simulink model "AdaptiveIDMF"  (R2022a)
settings: Solver=ode4  StartTime=0.0  StopTime=30  FixedStep=0.01  RelTol=1e-3
PostLoadFcn:
  | %Add subfolders to path
  | addpath('virtualworld');
InitFcn:
  | startScript;
values from neighbouring files (symbols this model uses):
  angularVelocity = [0 0 -0.01]    [startScript.m]
  angularVelocityforLanding = [0 0 0]    [startScript.m]
  dronestartlocation = [-1.5 0 4]    [startScript.m]
  Dstar = -0.5    [startScript.m]
  finalHoverHeight = 2.5    [startScript.m]
  helipadLocation = [14 0.6 5]    [startScript.m]
  linearVelocity = [5 0.05 1]    [startScript.m]
  linearVelocityforHover = [0.65 0.05 0.3]    [startScript.m]
  ypmin = yps(iypmin,:)    [hyperpred.m]
undefined symbols (not defined in the file or in its folder): fspecial, gcbh, Kanade, Lucas, Rec, SDTV, vrmfunc
libraries: visiontextngfix x10, visionconversions x9, vrlib x7, visionanalysis x7, slpidlib x4, sharedtransform x2, simulink x1
(part 2 of 3)

== system AdaptiveIDMF/ Optical Flow Algorithm for Obstacle Avoidance/Optical flow algorithm and PID Controller for landing/DronePositionEstimation.OpticalFlowAlgorithm_ ==
  note: If the output from the Sign block is Positive, drone should move towards the left side, i.e. V_y is Negative. Also, if the output from the Sign block is Negative, drone will move towwars the right side..ie, V_y is Positive.
  note: Steering Linear Velocities
  OpticalFlowDiff : Inport
  Action Port : ActionPort
      settings: CopyFcn=Stateflow.SLINSF.SimulinkMan.removeBlockPreDeleteFcn  PreDeleteFcn=Stateflow.SLINSF.SimulinkMan.unsafePredeleteFcn
  Constant : Constant  Value=uint32(zeros(50,2))
  Constant1 : Constant  Value=linearVelocity
  Constant3 : Constant  Value=-1
  Gain : Gain  Gain=[1 1 -1]
  Integrator2 : Integrator  InitialCondition=dronestartlocation
  Sign : Signum
  Switch1 : Switch  Criteria=u2 > Threshold  SaturateOnIntegerOverflow=off  InputSameDT=off
  PositionOutput : Outport
  detectedpoints : Outport  Port=2
      settings: VarSizeSig=Yes
  reset : Outport  Port=3
  wires:
  OpticalFlowDiff/1 -> Sign/1
  Constant1/1 -> Switch1/3, Gain/1  "[V_X V_Z V_Y]"
  Switch1/1 -> Integrator2/1
  Gain/1 -> Switch1/1  "[V_X V_Z -1*V_Y]"
  Constant/1 -> detectedpoints/1
  Sign/1 -> Switch1/2
  Integrator2/1 -> PositionOutput/1
  Constant3/1 -> reset/1

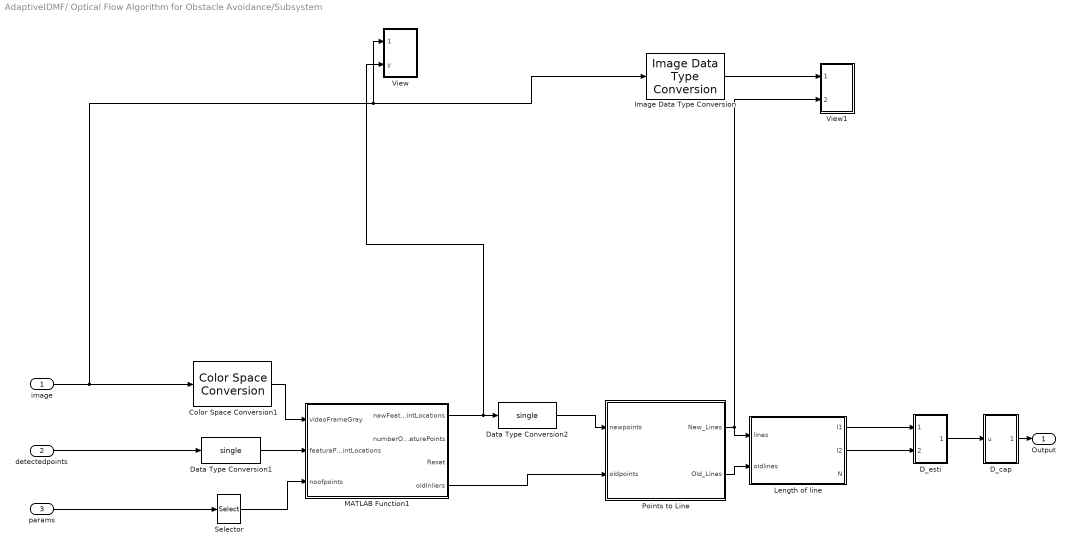
== system AdaptiveIDMF/ Optical Flow Algorithm for Obstacle Avoidance/Subsystem ==
  image : Inport
  detectedpoints : Inport  Port=2
  params : Inport  Port=3
  Color Space Conversion1 : visionconversions/Color Space  Conversion  conversion=Obsolete  conversionActive=R'G'B' to intensity  wp_str=D65  rec=Rec. 601 (SDTV)  sys=1125/60/2:1  imagePorts=One multidimensional signal
  D_cap : Subsystem
  D_esti : Subsystem
  Data Type Conversion1 : DataTypeConversion  OutDataTypeStr=single  SaturateOnIntegerOverflow=off  RndMeth=Floor
  Data Type Conversion2 : DataTypeConversion  OutDataTypeStr=single  SaturateOnIntegerOverflow=off  RndMeth=Floor
  Image Data Type Conversion : visionconversions/Image Data Type Conversion  outDT=single  isSigned=on  wordLen=16  numFracBits=0
      settings: SourceProductBaseCode=VP
  Length of line : MATLAB Function  TreatAsAtomicUnit=on
  MATLAB Function1 : MATLAB Function  TreatAsAtomicUnit=on
  Points to Line : MATLAB Function  TreatAsAtomicUnit=on
  Selector : Selector  InputPortWidth=6  IndexOptions=Index vector (dialog)  Indices=2  OutputSizes=1
  View : Subsystem
  View1 : Subsystem
  Output : Outport
  wires:
  Data Type Conversion1/1 -> MATLAB Function1/2(featurePointLocations)
  Color Space Conversion1/1 -> MATLAB Function1/1(videoFrameGray)
  MATLAB Function1/4(oldInliers) -> Points to Line/2(oldpoints)
  Points to Line/2(Old_Lines) -> Length of line/2(oldlines)
  params/1 -> Selector/1
  Selector/1 -> MATLAB Function1/3(noofpoints)
  Length of line/1(l1) -> D_esti/1(In1)
  Length of line/2(l2) -> D_esti/2(In2)
  D_esti/1(Out1) -> D_cap/1(u)
  D_cap/1(Out1) -> Output/1
  MATLAB Function1/1(newFeaturePointLocations) -> View/2(y), Data Type Conversion2/1
  Data Type Conversion2/1 -> Points to Line/1(newpoints)
  detectedpoints/1 -> Data Type Conversion1/1
  image/1 -> Image Data Type Conversion/1, View/1(d_camera), Color Space Conversion1/1
  Points to Line/1(New_Lines) -> View1/2(vel_Lines), Length of line/1(lines)
  Image Data Type Conversion/1 -> View1/1(camera_d)

== system AdaptiveIDMF/ Optical Flow Algorithm for Obstacle Avoidance/flowdiff ==
  image : Inport
  Delay1 : Delay  DelayLength=4
  FlowDifferences : MATLAB Function  TreatAsAtomicUnit=on
  Gain : Gain  Gain=1/10^3
  Sum1 : Sum  Inputs=+-
  Out1 : Outport
  Out2 : Outport  Port=2
  vleftflow : Outport  Port=3
  vrightflow : Outport  Port=4
  cmd : Outport  Port=5
  wires:
  Gain/1 -> Out2/1, Delay1/1, Sum1/1
  FlowDifferences/1(flowDifference) -> Gain/1
  Sum1/1 -> Out1/1
  FlowDifferences/3(vrightflow) -> vrightflow/1
  FlowDifferences/4(cmd) -> cmd/1
  Delay1/1 -> Sum1/2
  image/1 -> FlowDifferences/1(image)
  FlowDifferences/2(vleftflow) -> vleftflow/1

== system AdaptiveIDMF/ Optical Flow Algorithm for Obstacle Avoidance/flowdiff_down ==
  image : Inport
  Delay : Delay  DelayLength=10
  Delay2 : Delay  DelayLength=10
  FlowDifferences1 : MATLAB Function  TreatAsAtomicUnit=on
  FlowDifferences2 : MATLAB Function  TreatAsAtomicUnit=on
  Gain1 : Gain  Gain=1/10^3
  Gain2 : Gain  Gain=1/10^3
  Sum : Sum  Inputs=+-
  Sum2 : Sum  Inputs=+-
  ofd_up_d : Outport
  flowdiff_down : Outport  Port=2
  ofd_d : Outport  Port=3
  flowup_down : Outport  Port=4
  wires:
  image/1 -> FlowDifferences2/1(image), FlowDifferences1/1(image)
  Gain1/1 -> flowdiff_down/1, Sum/1, Delay/1  "flowdiff_down"
  Gain2/1 -> flowup_down/1, Delay2/1, Sum2/1  "flowup_down"
  FlowDifferences1/1(flowDifference) -> Gain1/1  "flowdiff_down"
  Delay/1 -> Sum/2
  FlowDifferences2/1(flowDifference) -> Gain2/1  "flowup_down"
  Sum2/1 -> ofd_up_d/1  "ofd_up_d"
  Delay2/1 -> Sum2/2
  Sum/1 -> ofd_d/1  "ofd_d"

== system AdaptiveIDMF/Optical Flow Lines Calculation/Optical Flow Lines ==
  vel.Values : Inport
  Optical Flow Lines : MATLAB Function  TreatAsAtomicUnit=on
  vel.Lines : Outport
  wires:
  Optical Flow Lines/1(vel_Lines) -> vel.Lines/1
  vel.Values/1 -> Optical Flow Lines/1(vel_Values)

== system AdaptiveIDMF/Optical Flow Lines Calculation/Optical Flow Lines1 ==
  vel.Values : Inport
  Optical Flow Lines : MATLAB Function  TreatAsAtomicUnit=on
  vel.Lines : Outport
  wires:
  Optical Flow Lines/1(vel_Lines) -> vel.Lines/1
  vel.Values/1 -> Optical Flow Lines/1(vel_Values)

== system AdaptiveIDMF/Optical Flow Lines Calculation1/D ==
  Clock : Clock
  Gain : Gain  Gain=5
  Memory : Memory
  Sum1 : Sum  Inputs=+-
  Out2 : Outport
  wires:
  Clock/1 -> Memory/1, Sum1/1
  Sum1/1 -> Gain/1
  Memory/1 -> Sum1/2
  Gain/1 -> Out2/1

== system AdaptiveIDMF/Optical Flow Lines Calculation1/View ==
  d_camera : Inport
  In2 : Inport  Port=2
  Data Type Conversion : DataTypeConversion  OutDataTypeStr=int32  SaturateOnIntegerOverflow=off  RndMeth=Floor
  Draw Markers1 : visiontextngfix/Draw Markers  shape=X-mark  size=3  fill=off  fillClrSource=Specify via dialog  display=User-specified value  intensity=200  color=[255 0 0]  opacity=0.6  viewport=Entire image  antialiasing=off  inType=Obsolete  imagePorts=One multidimensional signal  roundingMode=Floor  overflowMode=off  memoryMode=Specify word length  memoryWordLength=16  memoryFracLength=15  prodOutputMode=Binary point scaling  prodOutputWordLength=32  prodOutputFracLength=14
      settings: SourceProductBaseCode=VP
  points for ownline : VideoViewer  FigPos=[132 616 560 453]
  wires:
  In2/1 -> Data Type Conversion/1
  Draw Markers1/1 -> points for ownline/1
  d_camera/1 -> Draw Markers1/1
  Data Type Conversion/1 -> Draw Markers1/2

== system AdaptiveIDMF/Optical Flow Lines Calculation1/View1 ==
  In1 : Inport
  In2 : Inport  Port=2
  Data Type Conversion : DataTypeConversion  OutDataTypeStr=int32  SaturateOnIntegerOverflow=off  RndMeth=Floor
  Draw Shapes2 : visiontextngfix/Draw Shapes  shape=Lines  fill=off  lineWidth=1  fillClrSource=Specify via dialog  display=User-specified value  intensity=200  color=[255 255 0]  opacity=0.6  viewport=Entire image  antialiasing=off  inType=Obsolete  imagePorts=One multidimensional signal  roundingMode=Floor  overflowMode=off  memoryMode=Specify word length  memoryWordLength=16  prodOutputMode=Binary point scaling  prodOutputWordLength=32  prodOutputFracLength=14  memoryFracLength=15
  owncode lines : VideoViewer  FigPos=[594 703 418 304]
  wires:
  Draw Shapes2/1 -> owncode lines/1
  In1/1 -> Draw Shapes2/1
  Data Type Conversion/1 -> Draw Shapes2/2
  In2/1 -> Data Type Conversion/1

== system AdaptiveIDMF/ Optical Flow Algorithm for Obstacle Avoidance/Optical flow algorithm and PID Controller for landing/DronePositionEstimation.DroneLandingnoZ/Landing ==
  note: Steering Linear Velocities
  In1 : Inport
  D_est : Inport  Port=2
  linearVelocity : Inport  Port=3
  ypmin : Inport  Port=4
  Bus Creator1 : BusCreator  Inputs=3
  Constant : Constant  Value=linearVelocity
  Integrator2 : Integrator  InitialConditionSource=external  InitialCondition=dronestartlocation
  Manual Switch : ManualSwitch  CurrentSetting=0
  Manual Switch1 : ManualSwitch  CurrentSetting=0
  Selector2 : Selector  InputPortWidth=3  IndexOptions=Index vector (dialog)  Indices=[2]  OutputSizes=1
  Selector3 : Selector  InputPortWidth=3  IndexOptions=Index vector (dialog)  Indices=[3]  OutputSizes=1
  Selector4 : Selector  InputPortWidth=3  IndexOptions=Index vector (dialog)  Indices=[1]  OutputSizes=1
  Subsystem : Subsystem
  PositionOutput : Outport
  reset : Outport  Port=2
  wires:
  D_est/1 -> Subsystem/2(D_est)
  Selector4/1 -> Bus Creator1/1
  Selector3/1 -> Bus Creator1/3
  Subsystem/1(Z) -> Bus Creator1/2
  Bus Creator1/1 -> PositionOutput/1
  Selector2/1 -> Subsystem/1(InitialZ)
  Manual Switch/1 -> Integrator2/1  "[V_X V_Z -1*V_Y]"
  Constant/1 -> Manual Switch/1
  Integrator2/1 -> Manual Switch1/1
  linearVelocity/1 -> Manual Switch/2
  Manual Switch1/1 -> Selector4/1, Selector3/1, Selector2/1
  In1/1 -> Integrator2/2, Manual Switch1/2
  Subsystem/2(Output) -> reset/1
  ypmin/1 -> Subsystem/3(params)

== system AdaptiveIDMF/ Optical Flow Algorithm for Obstacle Avoidance/Optical flow algorithm and PID Controller for landing/DronePositionEstimation.DroneLandingnoZ/Subsystem ==
  Input : Inport
  Color Space Conversion1 : visionconversions/Color Space  Conversion  conversion=Obsolete  conversionActive=R'G'B' to intensity  wp_str=D65  rec=Rec. 601 (SDTV)  sys=1125/60/2:1  imagePorts=One multidimensional signal
  Corner Detection : visionanalysis/Corner Detection  method=Local intensity comparison (Rosen & Drummond)  factor=0.04  filter=fspecial('gaussian', [1 5], 1.5)  thrInten=0.1  thrAngle=157.5  output=Obsolete9b  outputInUse=Corner location  maxNum=50  thrMetric=0.005  neighborSize=[15 15]  isOutVarDim=off  roundingMode=Floor  overflowMode=off  firstCoeffMode=Specify word length  firstCoeffWordLength=16  firstCoeffFracLength=16  prodOutputMode=Binary point scaling  prodOutputWordLength=32  prodOutputFracLength=0  accumMode=Binary point scaling  accumWordLength=32  accumFracLength=0  memoryMode=Binary point scaling  memoryWordLength=32  memoryFracLength=0
      settings: SourceProductBaseCode=VP
  Output : Outport
  wires:
  Input/1 -> Color Space Conversion1/1
  Color Space Conversion1/1 -> Corner Detection/1
  Corner Detection/1 -> Output/1

== system AdaptiveIDMF/ Optical Flow Algorithm for Obstacle Avoidance/Subsystem/D_cap ==
  u : Inport
  Divide1 : Product  Inputs=*/
  Pre-proessing : Subsystem
  sumele : MATLAB Function  TreatAsAtomicUnit=on
  Out1 : Outport
  wires:
  sumele/2(n1) -> Divide1/2
  Divide1/1 -> Pre-proessing/1(Dca)  "Dca"
  sumele/1(y1) -> Divide1/1
  Pre-proessing/1(Out1) -> Out1/1
  u/1 -> sumele/1(u)

== system AdaptiveIDMF/ Optical Flow Algorithm for Obstacle Avoidance/Subsystem/D_esti ==
  In1 : Inport
  In2 : Inport  Port=2
  Constant : Constant  Value=0.1
  Divide : Product  Inputs=*//
  Sum : Sum  Inputs=|-+
  Out1 : Outport
  wires:
  Sum/1 -> Divide/1
  Constant/1 -> Divide/3
  In2/1 -> Divide/2, Sum/2
  In1/1 -> Sum/1
  Divide/1 -> Out1/1

== system AdaptiveIDMF/ Optical Flow Algorithm for Obstacle Avoidance/Subsystem/View ==
  d_camera : Inport
  y : Inport  Port=2
  Data Type Conversion : DataTypeConversion  OutDataTypeStr=int32  SaturateOnIntegerOverflow=off  RndMeth=Floor
  Draw Markers1 : visiontextngfix/Draw Markers  shape=X-mark  size=3  fill=off  fillClrSource=Specify via dialog  display=User-specified value  intensity=200  color=[255 0 0]  opacity=0.6  viewport=Entire image  antialiasing=off  inType=Obsolete  imagePorts=One multidimensional signal  roundingMode=Floor  overflowMode=off  memoryMode=Specify word length  memoryWordLength=16  memoryFracLength=15  prodOutputMode=Binary point scaling  prodOutputWordLength=32  prodOutputFracLength=14
      settings: SourceProductBaseCode=VP
  points from new : VideoViewer  FigPos=[1018 724 504 408]
  wires:
  y/1 -> Data Type Conversion/1
  Draw Markers1/1 -> points from new/1
  d_camera/1 -> Draw Markers1/1
  Data Type Conversion/1 -> Draw Markers1/2

== system AdaptiveIDMF/ Optical Flow Algorithm for Obstacle Avoidance/Subsystem/View1 ==
  camera_d : Inport
  vel_Lines : Inport  Port=2
  Detected lines : VideoViewer  FigPos=[540 661 571 460]
  Draw Shapes2 : visiontextngfix/Draw Shapes  shape=Lines  fill=off  lineWidth=1  fillClrSource=Specify via dialog  display=User-specified value  intensity=200  color=[255 255 0]  opacity=0.6  viewport=Entire image  antialiasing=off  inType=Obsolete  imagePorts=One multidimensional signal  roundingMode=Floor  overflowMode=off  memoryMode=Specify word length  memoryWordLength=16  prodOutputMode=Binary point scaling  prodOutputWordLength=32  prodOutputFracLength=14  memoryFracLength=15
  wires:
  camera_d/1 -> Draw Shapes2/1
  vel_Lines/1 -> Draw Shapes2/2
  Draw Shapes2/1 -> Detected lines/1

== system AdaptiveIDMF/ Optical Flow Algorithm for Obstacle Avoidance/Optical flow algorithm and PID Controller for landing/DronePositionEstimation.DroneLandingnoZ/Landing/Subsystem ==
  InitialZ : Inport
  D_est : Inport  Port=2
  params : Inport  Port=3
  Subsystem : Subsystem
  Subsystem1 : Subsystem
  Z : Outport
  Output : Outport  Port=2
  wires:
  InitialZ/1 -> Subsystem/1(InitialZ), Subsystem1/1(InitialZ)
  D_est/1 -> Subsystem/2(D_est)
  Subsystem/1(Z) -> Subsystem1/2(calcZ)
  Subsystem/2(resetp) -> Subsystem1/3(resetp)
  Subsystem1/1(Z) -> Z/1
  Subsystem1/2(Output) -> Output/1
  params/1 -> Subsystem1/4(params), Subsystem/3(params)

== system AdaptiveIDMF/ Optical Flow Algorithm for Obstacle Avoidance/Subsystem/D_cap/Pre-proessing ==
  Dca : Inport
  Constant1 : Constant  Value=0
  IsNaN : RelationalOperator  Operator=isNaN  OutDataTypeStr=boolean  RndMeth=Simplest  InputSameDT=off
  Rate Transition : RateTransition  OutPortSampleTime=0.01
  Switch : Switch  Threshold=1  SaturateOnIntegerOverflow=off  InputSameDT=off
  Out1 : Outport
  wires:
  Constant1/1 -> Switch/1
  Dca/1 -> Switch/3, IsNaN/1
  Switch/1 -> Rate Transition/1
  IsNaN/1 -> Switch/2
  Rate Transition/1 -> Out1/1

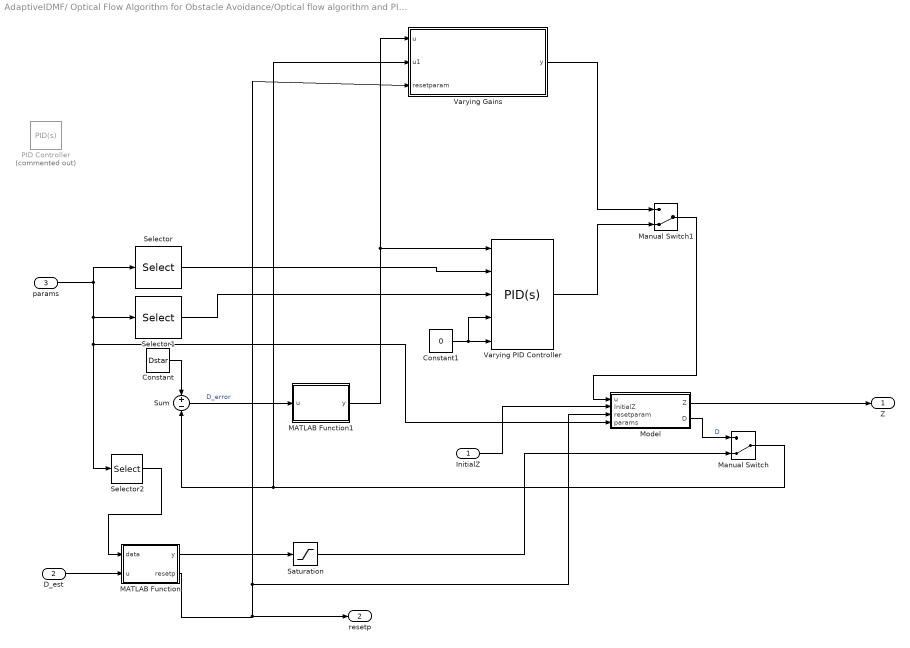
== system AdaptiveIDMF/ Optical Flow Algorithm for Obstacle Avoidance/Optical flow algorithm and PID Controller for landing/DronePositionEstimation.DroneLandingnoZ/Landing/Subsystem/Subsystem ==
  InitialZ : Inport
  D_est : Inport  Port=2
  params : Inport  Port=3
  Constant : Constant  Value=Dstar
  Constant1 : Constant  Value=0
  MATLAB Function : MATLAB Function  TreatAsAtomicUnit=on
  MATLAB Function1 : MATLAB Function  TreatAsAtomicUnit=on
  Manual Switch : ManualSwitch  CurrentSetting=0
  Manual Switch1 : ManualSwitch  CurrentSetting=0
  Model : Subsystem
  PID Controller : slpidlib/PID Controller  Commented=on  Controller=PID  Form=Parallel  TimeDomain=Continuous-time  UseExternalTs=off  SampleTime=-1  IntegratorMethod=Forward Euler  FilterMethod=Forward Euler  ControllerParametersSource=internal  P=1  I=1  UseKiTs=off  D=0  N=100  UseFilter=on  TunerSelectOption=Transfer Function Based (PID Tuner App)  InitialConditionSource=internal  InitialConditionForIntegrator=0  InitialConditionForFilter=0  DifferentiatorICPrevScaledInput=0  ExternalReset=none  TrackingMode=off  Kt=1  LimitOutput=off  SatLimitsSource=internal  UpperSaturationLimit=inf  LowerSaturationLimit=-inf  LinearizeAsGain=on  AntiWindupMode=none  Kb=1  POutMin=[]  POutMax=[]  IOutMin=[]  IOutMax=[]  DOutMin=[]  DOutMax=[]  NOutMin=[]  NOutMax=[]  SumOutMin=[]  SumOutMax=[]  SaturationOutMin=[]  SaturationOutMax=[]  PParamMin=[]  PParamMax=[]  IParamMin=[]  IParamMax=[]  DParamMin=[]  DParamMax=[]  NParamMin=[]  NParamMax=[]  KbParamMin=[]  KbParamMax=[]  KtParamMin=[]  KtParamMax=[]  KbOutMin=[]  KbOutMax=[]  KtOutMin=[]  KtOutMax=[]  IntegratorOutMin=[]  IntegratorOutMax=[]  FilterOutMin=[]  FilterOutMax=[]  SumI1OutMin=[]  SumI1OutMax=[]  SumI2OutMin=[]  SumI2OutMax=[]  SumI3OutMin=[]  SumI3OutMax=[]  SumI4OutMin=[]  SumI4OutMax=[]  SumDOutMin=[]  SumDOutMax=[]  DifferentiatorOutMin=[]  DifferentiatorOutMax=[]  FilterDiffOutCoefMin=[]  FilterDiffOutCoefMax=[]  ReciprocalOutMin=[]  ReciprocalOutMax=[]  SumDenOutMin=[]  SumDenOutMax=[]  SumNumOutMin=[]  SumNumOutMax=[]  DivideOutMin=[]  DivideOutMax=[]  UdiffTsProdOutMin=[]  UdiffTsProdOutMax=[]  NTsProdOutMin=[]  NTsProdOutMax=[]  UintegralTsProdOutMin=[]  UintegralTsProdOutMax=[]  UngainTsProdOutMin=[]  UngainTsProdOutMax=[]  IntegratorContinuousStateAttributes=''  IntegratorStateMustResolveToSignalObject=off  IntegratorRTWStateStorageClass=Auto  FilterContinuousStateAttributes=''  FilterStateMustResolveToSignalObject=off  FilterRTWStateStorageClass=Auto  ParallelPVariant=InternalParameters  IdealPVariant=Disabled  IVariant=InternalParameters  DVariant=InternalParameters  IntegratorVariant=Continuous  SatVariant=Disabled  AWVariant=Passthrough  PCopyVariant=Disabled  TRVariant=Disabled  FdbkBlocksVariant=Forward  IdealPFdbkVariant=Disabled  SatFdbkVariant=Disabled  DerivativeFilterVariant=ContFilter  NVariant=InternalParameters  NCopyVariant=Disabled  FilterICVariant=InternalICsFilter  IntegratorICVariant=InternalICs  ExternalResetVariant=Disabled  TRSumVariant=Passthrough  SumFdbkVariant=Disabled  SumVariant=Sum_PID  TsampFilterVariant=InternalTs  TsampNgainVariant=Passthrough  TsampIntegralVariant=Passthrough  ExternalSaturationOutDataTypeStr=Inherit: Same as second input  aMode=0
  Saturation : Saturate  UpperLimit=1  LowerLimit=-1
  Selector : Selector  InputPortWidth=6  IndexOptions=Index vector (dialog)  Indices=3  OutputSizes=1
  Selector1 : Selector  InputPortWidth=6  IndexOptions=Index vector (dialog)  Indices=4  OutputSizes=1
  Selector2 : Selector  InputPortWidth=6  IndexOptions=Index vector (dialog)  Indices=5  OutputSizes=1
  Sum : Sum  Inputs=+-
  Varying Gains : Subsystem
  Varying PID Controller : slpidlib/PID Controller  Controller=PID  Form=Parallel  TimeDomain=Continuous-time  UseExternalTs=off  SampleTime=-1  IntegratorMethod=Forward Euler  FilterMethod=Forward Euler  ControllerParametersSource=external  P=1  I=1  UseKiTs=off  D=0  N=100  UseFilter=on  TunerSelectOption=Transfer Function Based (PID Tuner App)  InitialConditionSource=internal  InitialConditionForIntegrator=0  InitialConditionForFilter=0  DifferentiatorICPrevScaledInput=0  ExternalReset=none  TrackingMode=off  Kt=1  LimitOutput=off  SatLimitsSource=internal  UpperSaturationLimit=inf  LowerSaturationLimit=-inf  LinearizeAsGain=on  AntiWindupMode=none  Kb=1  POutMin=[]  POutMax=[]  IOutMin=[]  IOutMax=[]  DOutMin=[]  DOutMax=[]  NOutMin=[]  NOutMax=[]  SumOutMin=[]  SumOutMax=[]  SaturationOutMin=[]  SaturationOutMax=[]  PParamMin=[]  PParamMax=[]  IParamMin=[]  IParamMax=[]  DParamMin=[]  DParamMax=[]  NParamMin=[]  NParamMax=[]  KbParamMin=[]  KbParamMax=[]  KtParamMin=[]  KtParamMax=[]  KbOutMin=[]  KbOutMax=[]  KtOutMin=[]  KtOutMax=[]  IntegratorOutMin=[]  IntegratorOutMax=[]  FilterOutMin=[]  FilterOutMax=[]  SumI1OutMin=[]  SumI1OutMax=[]  SumI2OutMin=[]  SumI2OutMax=[]  SumI3OutMin=[]  SumI3OutMax=[]  SumI4OutMin=[]  SumI4OutMax=[]  SumDOutMin=[]  SumDOutMax=[]  DifferentiatorOutMin=[]  DifferentiatorOutMax=[]  FilterDiffOutCoefMin=[]  FilterDiffOutCoefMax=[]  ReciprocalOutMin=[]  ReciprocalOutMax=[]  SumDenOutMin=[]  SumDenOutMax=[]  SumNumOutMin=[]  SumNumOutMax=[]  DivideOutMin=[]  DivideOutMax=[]  UdiffTsProdOutMin=[]  UdiffTsProdOutMax=[]  NTsProdOutMin=[]  NTsProdOutMax=[]  UintegralTsProdOutMin=[]  UintegralTsProdOutMax=[]  UngainTsProdOutMin=[]  UngainTsProdOutMax=[]  IntegratorContinuousStateAttributes=''  IntegratorStateMustResolveToSignalObject=off  IntegratorRTWStateStorageClass=Auto  FilterContinuousStateAttributes=''  FilterStateMustResolveToSignalObject=off  FilterRTWStateStorageClass=Auto  ParallelPVariant=ExternalParameters  IdealPVariant=Disabled  IVariant=ExternalParameters  DVariant=ExternalParameters  IntegratorVariant=Continuous  SatVariant=Disabled  AWVariant=Passthrough  PCopyVariant=Disabled  TRVariant=Disabled  FdbkBlocksVariant=Forward  IdealPFdbkVariant=Disabled  SatFdbkVariant=Disabled  DerivativeFilterVariant=ContFilter  NVariant=ExternalParameters  NCopyVariant=Disabled  FilterICVariant=InternalICsFilter  IntegratorICVariant=InternalICs  ExternalResetVariant=Disabled  TRSumVariant=Passthrough  SumFdbkVariant=Disabled  SumVariant=Sum_PID  TsampFilterVariant=InternalTs  TsampNgainVariant=Passthrough  TsampIntegralVariant=Passthrough  ExternalSaturationOutDataTypeStr=Inherit: Same as second input  aMode=0
  Z : Outport
  resetp : Outport  Port=2
  wires:
  Sum/1 -> MATLAB Function1/1(u)  "D_error"
  Model/2(D) -> Manual Switch/1  "D"
  Model/1(Z) -> Z/1
  MATLAB Function1/1(y) -> Varying Gains/1(u), Varying PID Controller/1
  InitialZ/1 -> Model/2(InitialZ)
  Constant/1 -> Sum/1
  Manual Switch/1 -> Varying Gains/2(u1), Sum/2
  D_est/1 -> MATLAB Function/2(u)
  MATLAB Function/1(y) -> Saturation/1
  Saturation/1 -> Manual Switch/2
  Manual Switch1/1 -> Model/1(u)
  Varying Gains/1(y) -> Manual Switch1/1
  Varying PID Controller/1 -> Manual Switch1/2
  Selector/1 -> Varying PID Controller/2
  Selector1/1 -> Varying PID Controller/3
  Constant1/1 -> Varying PID Controller/4, Varying PID Controller/5
  params/1 -> Selector2/1, Model/4(params), Selector1/1, Selector/1
  Selector2/1 -> MATLAB Function/1(data)
  MATLAB Function/2(resetp) -> resetp/1, Varying Gains/3(resetparam), Model/3(resetparam)

== system AdaptiveIDMF/ Optical Flow Algorithm for Obstacle Avoidance/Optical flow algorithm and PID Controller for landing/DronePositionEstimation.DroneLandingnoZ/Landing/Subsystem/Subsystem1 ==
  InitialZ : Inport
  calcZ : Inport  Port=2
  resetp : Inport  Port=3
  params : Inport  Port=4
  Compare To Constant : simulink/Logic and Bit Operations/Compare To Constant  relop=>  const=0  OutDataTypeStr=boolean
  First Order Hold : FirstOrderHold  InitialOutput=finalHoverHeight  ErrorTolerance=inf  AllowContinuousInput=on
  MATLAB Function : MATLAB Function  TreatAsAtomicUnit=on
  MATLAB Function1 : MATLAB Function  Commented=on  TreatAsAtomicUnit=on
  Selector : Selector  InputPortWidth=6  IndexOptions=Index vector (dialog)  Indices=5  OutputSizes=1
  Stop Simulation : Stop
  Z : Outport
  Output : Outport  Port=2
  wires:
  resetp/1 -> Output/1, MATLAB Function/1(resetp)
  InitialZ/1 -> MATLAB Function/3(currentz)
  calcZ/1 -> MATLAB Function/2(calcz)
  MATLAB Function/2(stp) -> Compare To Constant/1
  Compare To Constant/1 -> Stop Simulation/1
  MATLAB Function/3(x1) -> ?
  MATLAB Function/1(opz) -> First Order Hold/1
  First Order Hold/1 -> Z/1
  Selector/1 -> MATLAB Function/4(resetparam)
  params/1 -> Selector/1

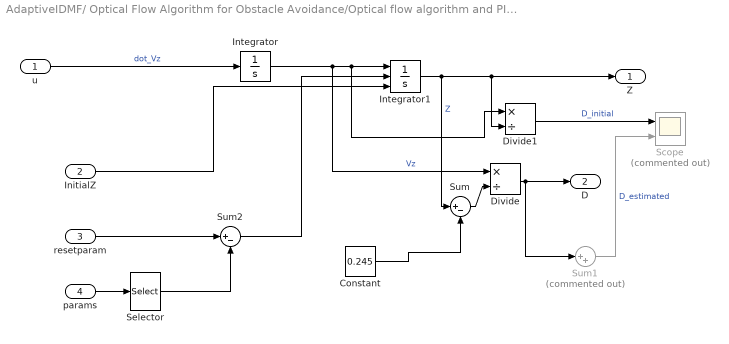
== system AdaptiveIDMF/ Optical Flow Algorithm for Obstacle Avoidance/Optical flow algorithm and PID Controller for landing/DronePositionEstimation.DroneLandingnoZ/Landing/Subsystem/Subsystem/Model ==
  u : Inport
  InitialZ : Inport  Port=2
  resetparam : Inport  Port=3
  params : Inport  Port=4
  Constant : Constant  Value=0.245
  Divide : Product  Inputs=*/
  Divide1 : Product  Inputs=*/
  Integrator : Integrator  InitialCondition=linearVelocityforHover(2)
  Integrator1 : Integrator  ExternalReset=falling  InitialConditionSource=external
  Scope : Scope  Commented=on  NumInputPorts=2
  Selector : Selector  InputPortWidth=6  IndexOptions=Index vector (dialog)  Indices=5  OutputSizes=1
  Sum : Sum  Inputs=|+-
  Sum1 : Sum  Commented=on  Inputs=|++
  Sum2 : Sum  Inputs=|+-
  Z : Outport
  D : Outport  Port=2
  wires:
  u/1 -> Integrator/1  "dot_Vz"
  Integrator/1 -> Divide/1, Divide1/1, Integrator1/1  "Vz"
  Integrator1/1 -> Sum/1, Divide1/2, Z/1  "Z"
  Divide/1 -> Sum1/1, D/1
  InitialZ/1 -> Integrator1/3
  Constant/1 -> Sum/2
  Sum/1 -> Divide/2
  Sum1/1 -> Scope/2  "D_estimated"
  Divide1/1 -> Scope/1  "D_initial"
  Sum2/1 -> Integrator1/2
  resetparam/1 -> Sum2/1
  params/1 -> Selector/1
  Selector/1 -> Sum2/2

== system AdaptiveIDMF/ Optical Flow Algorithm for Obstacle Avoidance/Optical flow algorithm and PID Controller for landing/DronePositionEstimation.DroneLandingnoZ/Landing/Subsystem/Subsystem/Varying Gains ==
  u : Inport
  u1 : Inport  Port=2
  resetparam : Inport  Port=3
  Constant1 : Constant  Value=9
  Constant2 : Constant  Value=0
  Varying PID Controller : slpidlib/PID Controller  Controller=PID  Form=Parallel  TimeDomain=Continuous-time  UseExternalTs=off  SampleTime=-1  IntegratorMethod=Forward Euler  FilterMethod=Forward Euler  ControllerParametersSource=external  P=1  I=1  UseKiTs=off  D=0  N=100  UseFilter=on  TunerSelectOption=Transfer Function Based (PID Tuner App)  InitialConditionSource=internal  InitialConditionForIntegrator=0  InitialConditionForFilter=0  DifferentiatorICPrevScaledInput=0  ExternalReset=none  TrackingMode=off  Kt=1  LimitOutput=off  SatLimitsSource=internal  UpperSaturationLimit=inf  LowerSaturationLimit=-inf  LinearizeAsGain=on  AntiWindupMode=none  Kb=1  POutMin=[]  POutMax=[]  IOutMin=[]  IOutMax=[]  DOutMin=[]  DOutMax=[]  NOutMin=[]  NOutMax=[]  SumOutMin=[]  SumOutMax=[]  SaturationOutMin=[]  SaturationOutMax=[]  PParamMin=[]  PParamMax=[]  IParamMin=[]  IParamMax=[]  DParamMin=[]  DParamMax=[]  NParamMin=[]  NParamMax=[]  KbParamMin=[]  KbParamMax=[]  KtParamMin=[]  KtParamMax=[]  KbOutMin=[]  KbOutMax=[]  KtOutMin=[]  KtOutMax=[]  IntegratorOutMin=[]  IntegratorOutMax=[]  FilterOutMin=[]  FilterOutMax=[]  SumI1OutMin=[]  SumI1OutMax=[]  SumI2OutMin=[]  SumI2OutMax=[]  SumI3OutMin=[]  SumI3OutMax=[]  SumI4OutMin=[]  SumI4OutMax=[]  SumDOutMin=[]  SumDOutMax=[]  DifferentiatorOutMin=[]  DifferentiatorOutMax=[]  FilterDiffOutCoefMin=[]  FilterDiffOutCoefMax=[]  ReciprocalOutMin=[]  ReciprocalOutMax=[]  SumDenOutMin=[]  SumDenOutMax=[]  SumNumOutMin=[]  SumNumOutMax=[]  DivideOutMin=[]  DivideOutMax=[]  UdiffTsProdOutMin=[]  UdiffTsProdOutMax=[]  NTsProdOutMin=[]  NTsProdOutMax=[]  UintegralTsProdOutMin=[]  UintegralTsProdOutMax=[]  UngainTsProdOutMin=[]  UngainTsProdOutMax=[]  IntegratorContinuousStateAttributes=''  IntegratorStateMustResolveToSignalObject=off  IntegratorRTWStateStorageClass=Auto  FilterContinuousStateAttributes=''  FilterStateMustResolveToSignalObject=off  FilterRTWStateStorageClass=Auto  ParallelPVariant=ExternalParameters  IdealPVariant=Disabled  IVariant=ExternalParameters  DVariant=ExternalParameters  IntegratorVariant=Continuous  SatVariant=Disabled  AWVariant=Passthrough  PCopyVariant=Disabled  TRVariant=Disabled  FdbkBlocksVariant=Forward  IdealPFdbkVariant=Disabled  SatFdbkVariant=Disabled  DerivativeFilterVariant=ContFilter  NVariant=ExternalParameters  NCopyVariant=Disabled  FilterICVariant=InternalICsFilter  IntegratorICVariant=InternalICs  ExternalResetVariant=Disabled  TRSumVariant=Passthrough  SumFdbkVariant=Disabled  SumVariant=Sum_PID  TsampFilterVariant=InternalTs  TsampNgainVariant=Passthrough  TsampIntegralVariant=Passthrough  ExternalSaturationOutDataTypeStr=Inherit: Same as second input  aMode=0
  variable P : Subsystem
  y : Outport
  wires:
  Constant2/1 -> Varying PID Controller/5, Varying PID Controller/4
  u/1 -> Varying PID Controller/1
  Constant1/1 -> Varying PID Controller/3
  u1/1 -> variable P/1(u)
  variable P/1(Out1) -> Varying PID Controller/2  "P"
  resetparam/1 -> variable P/2(resetparam)
  Varying PID Controller/1 -> y/1

== system AdaptiveIDMF/ Optical Flow Algorithm for Obstacle Avoidance/Optical flow algorithm and PID Controller for landing/DronePositionEstimation.DroneLandingnoZ/Landing/Subsystem/Subsystem/Varying Gains/variable P ==
  u : Inport
  resetparam : Inport  Port=2
  Constant3 : Constant  Value=2
  MATLAB Function : MATLAB Function  TreatAsAtomicUnit=on
  Sum1 : Sum  Inputs=|++
  Out1 : Outport
  wires:
  Constant3/1 -> Sum1/1
  Sum1/1 -> Out1/1
  u/1 -> MATLAB Function/1(u)
  MATLAB Function/1(y) -> Sum1/2
  resetparam/1 -> MATLAB Function/2(resetparam)

== matlab function AdaptiveIDMF/Optical Flow Lines Calculation1/Optical Flow Lines3 ==
  settings: updateMethod=DISCRETE
  data: vel_Values input; vel_Lines output; scaleFactor input size=1
function vel_Lines=OpticalFlowLines(vel_Values, scaleFactor) 

% Generates the coordinate points of optical flow lines

persistent first_time;
persistent X;
persistent Y;
persistent RV;
persistent CV;
if isempty(first_time)
    first_time     = 1;
    %% user may change the following three parameters
    borderOffset   = 5;
    decimFactorRow = 5;
    decimFactorCol = 5;    
    %%
    [R C] = size(vel_Values);
    RV = borderOffset:decimFactorRow:(R-borderOffset);   
    CV = borderOffset:decimFactorCol:(C-borderOffset);
    [Y X] = meshgrid(CV,RV);
end

tmp = vel_Values(RV,CV);
tmp = tmp.*scaleFactor;
vel_Lines = [Y(:), X(:), Y(:)+real(tmp(:)),  X(:)+imag(tmp(:))];

== matlab function AdaptiveIDMF/ Optical Flow Algorithm for Obstacle Avoidance/flowdiff_down/FlowDifferences1 ==
  data: flowDifference output; image input
function flowDifference = calculatethedifference(image)

% Image Preprocessing
image = flip(image, 1);

% Image Width
width = size(image,2);

% Calculate optical flow on right-half and the left-half of the image
VLeftFlow = image(:, 1:width/2); 
VRightFlow = image(:, width/2:width);

% Sum to get the total Optical Flow on the right-half and on left-half
vleftflow = sum(VLeftFlow(:));
vrightflow = sum(VRightFlow(:));

% Find the difference of the flow between the two halves
flowDifference = (vleftflow - vrightflow);

% Steer in the direction that has less optical flow which implies less 
% obstacles

== stateflow chart AdaptiveIDMF/ Optical Flow Algorithm for Obstacle Avoidance/Optical flow algorithm and PID Controller for landing ==
  settings: sampleTime=0.01
  state DronePositionEstimation [parallel]
    settings: executionOrder=1
    note: Controller for position is divided into three states:
        | Navigate left right based on optical flow lines
        | 2. Navigate the drone to hover over helipadLocation using PID controller
        | 3. Landing on the helipad from the height the drone was hovering at
    state DroneHover
    state OpticalFlowAlgorithm_
    state DroneLandingnoZ
    state DroneLanding2
    state DroneHover1
    (default) -> DronePositionEstimation.OpticalFlowAlgorithm_
    (junction 211) -> DroneHover
    DroneHover1 -> (junction 211) : [abs(xLocation-14) <= 0.3]
    DroneHover -> (junction 209) : [abs(PositionfromSensor(3)-5) <= 0.2...
        | && abs(xLocation-14) <= 0.1]
    (junction 209) -> DroneLandingnoZ
    DronePositionEstimation.OpticalFlowAlgorithm_ -> (junction 243) : [xLocation > 13]
    (junction 243) -> DroneLanding2
    DroneLanding2 -> DroneHover1 : [abs(zLocation-finalHoverHeight) <= 0.005]
  state ControlAlgorithm_ [parallel] [commented out]
  state DroneLanding [parallel] [commented out]
  state DroneLanding1 [parallel] [commented out]
  state DroneLanding_ [parallel] [commented out]
  note: condition to switch to drone landing:
      |
      | [abs(yLocation-helipadLocation(3)) <= delta...
      | && abs(xLocation-helipadLocation(1)) <= delta]
      | [abs(zLocation-finalHoverHeight) <= 0.05]
      | ofd>470 for -1.5 0 0
      | [abs(ofd_d)>0.4]
      | [ofd<-1 && xLocation > switchingXLimit]
      | [ofd_d>2.2]
      | [abs(ofd_d)>2.5] for -1.5 0 0
      | [abs(ofd_d)>1.9] for -1.5 0 4
      | [abs(ofd_d)<=0.006 && abs(ofd_up_d)<=0.04]
      | [abs(ofd_d)<=0.01 && abs(ofd_up_d)<=0.6]
      |
      |
      | [abs(data)-abs(flowDifference)<=0.05]
  state DroneOrientationEstimation [parallel]
    settings: executionOrder=2
    note: Controller for orientation is divided into two parts:
        | Navigate left right based on optical flow lines
        | Constant angular velocity to move to helipadLocation
    state OpticalFlowAlgorithm_
    state ControlAlgorithm_
    (default) -> DroneOrientationEstimation.OpticalFlowAlgorithm_
    DroneOrientationEstimation.OpticalFlowAlgorithm_ -> (junction 133) : [ofd>3 && xLocation > switchingXLimit]
    (junction 133) -> DroneOrientationEstimation.ControlAlgorithm_ : after(0.01,sec)
  note: for clear helipad:
      | [abs(flowup_down)<=0.115 && abs(flowdiff_down)<=0.035]
      | after(1.25,sec)
      |
      | for concentric helipad:
      | [abs(flowup_down)<=0.33 && abs(flowdiff_down)<=0.22]
      | ofd<-1000 &&
      | [abs(ofd_d)>1.9]
      |
      | [abs(ofd_d) <= 1.2...
      | && abs(ofd_up_d) <= 0.1]
      |
      | [abs(flowdiff_down) <= 0.04...
      | && abs(flowup_down) <= 0.06]
      |
      | abs(PositionfromSensor(3)-5) <= 0.1...
      | && abs(xLocation-14) <= 0.1
  data: sf_internal_action_state_placeholder_data local double size=1 =0; sf_internal_action_state_placeholder_data local double size=1 =0; sf_internal_action_state_placeholder_data local double size=1 =0; sf_internal_action_state_placeholder_data local double size=1 =0; sf_internal_action_state_placeholder_data local double size=1 =0; sf_internal_action_state_placeholder_data local double size=1 =0; sf_internal_action_state_placeholder_data local double size=1 =0; sf_internal_action_state_placeholder_data local double size=1 =0; sf_internal_action_state_placeholder_data local double size=1 =0; sf_internal_action_state_placeholder_data local double size=1 =0; sf_internal_action_state_placeholder_data local double size=1 =0; params input size=[1,6]; OpticalFlowDiff input; D_est input; ofd_up_d input; OrientationOutput output; zLocation input; PositionfromSensor input double; PositionOutput output; InitialCondition input; switchingXLimit local double; flowdiff_down input; finalHoverHeight input; xLocation input; camera_d input; ofd input; ofd_d input; flowup_down input; detectedpoints output size=[50 2]; reset output; DroneLandingnoZ1 output boolean; linearVelocity input

== matlab function AdaptiveIDMF/Optical Flow Lines Calculation/Optical Flow Lines1/Optical Flow Lines ==
  data: vel_Values input; vel_Lines output; scaleFactor parameter size=1
function vel_Lines=OpticalFlowLines(vel_Values, scaleFactor) 

% Generates the coordinate points of optical flow lines

persistent first_time;
persistent X;
persistent Y;
persistent RV;
persistent CV;
if isempty(first_time)
    first_time     = 1;
    %% user may change the following three parameters
    borderOffset   = 5;
    decimFactorRow = 5;
    decimFactorCol = 5;    
    %%
    [R C] = size(vel_Values);
    RV = borderOffset:decimFactorRow:(R-borderOffset);   
    CV = borderOffset:decimFactorCol:(C-borderOffset);
    [Y X] = meshgrid(CV,RV);
end

tmp = vel_Values(RV,CV);
tmp = tmp.*scaleFactor;
vel_Lines = [Y(:), X(:), Y(:)+real(tmp(:)), X(:)+imag(tmp(:))];

== matlab function AdaptiveIDMF/Optical Flow Lines Calculation1/Optical Flow Lines2 ==
  settings: updateMethod=DISCRETE
  data: vel_Values input; vel_Lines output; scaleFactor input size=1
function vel_Lines=OpticalFlowLines(vel_Values, scaleFactor) 

% Generates the coordinate points of optical flow lines

persistent first_time;
persistent X;
persistent Y;
persistent RV;
persistent CV;
if isempty(first_time)
    first_time     = 1;
    %% user may change the following three parameters
    borderOffset   = 5;
    decimFactorRow = 5;
    decimFactorCol = 5;    
    %%
    [R C] = size(vel_Values);
    RV = borderOffset:decimFactorRow:(R-borderOffset);   
    CV = borderOffset:decimFactorCol:(C-borderOffset);
    [Y X] = meshgrid(CV,RV);
end

tmp = vel_Values(RV,CV);
tmp = tmp.*scaleFactor;
vel_Lines = [Y(:), X(:), Y(:)+real(tmp(:)),  X(:)+imag(tmp(:))];

== matlab function AdaptiveIDMF/Optical Flow Lines Calculation/Optical Flow Lines/Optical Flow Lines ==
  data: vel_Values input; vel_Lines output; scaleFactor parameter size=1
function vel_Lines=OpticalFlowLines(vel_Values, scaleFactor) 

% Generates the coordinate points of optical flow lines

persistent first_time;
persistent X;
persistent Y;
persistent RV;
persistent CV;
if isempty(first_time)
    first_time     = 1;
    %% user may change the following three parameters
    borderOffset   = 5;
    decimFactorRow = 5;
    decimFactorCol = 5;    
    %%
    [R C] = size(vel_Values);
    RV = borderOffset:decimFactorRow:(R-borderOffset);   
    CV = borderOffset:decimFactorCol:(C-borderOffset);
    [Y X] = meshgrid(CV,RV);
end

tmp = vel_Values(RV,CV);
tmp = tmp.*scaleFactor;
vel_Lines = [Y(:), X(:), Y(:)+real(tmp(:)), X(:)+imag(tmp(:))];

== matlab function AdaptiveIDMF/ Optical Flow Algorithm for Obstacle Avoidance/Optical flow algorithm and PID Controller for landing/DronePositionEstimation.DroneLandingnoZ/Landing/Subsystem/Subsystem1/MATLAB Function ==
  settings: updateMethod=DISCRETE
  data: resetp input; opz output; calcz input; currentz input; stp output; x1 output; s output; resetparam input
function [opz,stp,x1,s] = fcn(resetp,calcz,currentz,resetparam)

persistent zval;
persistent stop;
persistent x;
persistent sl;
if isempty(zval)
    zval=calcz;
end
if isempty(stop)
    stop=0;
end
if isempty(x)
    x=0;
end
if isempty(sl)
    sl=0;
end
if resetp >resetparam
    if ((zval-x)<=0.4)
            x=x-0.005;
            opz=x;
            sl=sl+1;
    else 
        stop =1;
        opz=x;
    end
else 
    if zval~=x && x~=0
        zval=x;
        opz=x;
    else
    zval=calcz;
    opz=zval;
    x=zval;
    end
end
stp=stop;
x1=x;
s=sl;

== matlab function AdaptiveIDMF/ Optical Flow Algorithm for Obstacle Avoidance/flowdiff/FlowDifferences ==
  data: flowDifference output; vleftflow output; vrightflow output; cmd output; image input
function [flowDifference,vleftflow, vrightflow,cmd] = calculatethedifference(image)

% Image Preprocessing
image = flip(image, 1);

% Image Width
width = size(image,2);

% Calculate optical flow on right-half and the left-half of the image
VLeftFlow = image(:, 1:width/2); 
VRightFlow = image(:, width/2:width);

% Sum to get the total Optical Flow on the right-half and on left-half
vleftflow = sum(VLeftFlow(:));
vrightflow = sum(VRightFlow(:));

% Find the difference of the flow between the two halves
flowDifference = (vleftflow - vrightflow);

% Steer in the direction that has less optical flow which implies less 
% obstacles
if flowDifference>0
    cmd=uint8('Steering to Left ');
else
    cmd=uint8('Steering to Right');
end

== matlab function AdaptiveIDMF/ Optical Flow Algorithm for Obstacle Avoidance/flowdiff_down/FlowDifferences2 ==
  data: flowDifference output; image input
function flowDifference = calculatethedifference(image)

% Image Preprocessing
image = flip(image, 1);

% Image Width
% width = size(image,2);
length = size(image,1);

% Calculate optical flow on right-half and the left-half of the image
VUpFlow = image(length/2:length,:); 
VDownFlow = image(1:length/2, :);

% Sum to get the total Optical Flow on the right-half and on left-half
vupflow = sum(VUpFlow(:));
vdownflow = sum(VDownFlow(:));

% Find the difference of the flow between the two halves
flowDifference = (vupflow - vdownflow);

% Steer in the direction that has less optical flow which implies less 
% obstacles

== matlab function AdaptiveIDMF/Optical Flow Lines Calculation1/MATLAB Function1 ==
  data: points input; vel_Lines output int32 size=[50 4]; vel_points output int32 size=[50 2]
function [vel_Lines, vel_points]=OpticalFlowLines(points)
%persistent vel_Lines;

orderedpointsog = sortrows(points);
X = [];
Y = [];
shiftX = [];
shiftY=[];

%|| orderedpoints(i,1)==orderedpoints(i+1,1)+1 || orderedpoints(i,1)==orderedpoints(i+1,1)-1)
for i = 1:2:length(points)-1
    if i ==1 && orderedpointsog(i,1)==orderedpointsog(i+1,1) 
        X = [X ;orderedpointsog(i,1)];
        Y = [Y ;orderedpointsog(i,2)];
        shiftX = [shiftX ;orderedpointsog(i+1,1)];
        shiftY = [shiftY ;orderedpointsog(i+1,2)];
    else
        if i ~=1 && (orderedpointsog(i,1)==orderedpointsog(i+1,1)|| orderedpointsog(i,1)==orderedpointsog(i+1,1)+1 || orderedpointsog(i,1)==orderedpointsog(i+1,1)-1 ...
                || orderedpointsog(i,1)==orderedpointsog(i+1,1)+2 || orderedpointsog(i,1)==orderedpointsog(i+1,1)-2)
        X = [X ;orderedpointsog(i,1)];
        Y = [Y ;orderedpointsog(i,2)];
        shiftX = [shiftX ;orderedpointsog(i+1,1)];
        shiftY = [shiftY ;orderedpointsog(i+1,2)];
        
        elseif i~=1 &&  (orderedpointsog(i,1)==orderedpointsog(i-1,1)|| orderedpointsog(i,1)==orderedpointsog(i-1,1)+1 || orderedpointsog(i,1)==orderedpointsog(i-1,1)-1 ...
                || orderedpointsog(i,1)==orderedpointsog(i-1,1)+2 || orderedpointsog(i,1)==orderedpointsog(i-1,1)-2)
        X = [X ;orderedpointsog(i,1)];
        Y = [Y ;orderedpointsog(i,2)];
        shiftX = [shiftX ;orderedpointsog(i-1,1)];
        shiftY = [shiftY ;orderedpointsog(i-1,2)];
    end
   end


end
vel_points = [X(:), Y(:); shiftX(:),  shiftY(:) ];
vel_Lines = [X(:), Y(:), shiftX(:),  shiftY(:)];

== matlab function AdaptiveIDMF/ Optical Flow Algorithm for Obstacle Avoidance/Optical flow algorithm and PID Controller for landing/DronePositionEstimation.DroneLandingnoZ/Landing/Subsystem/Subsystem/MATLAB Function1 ==
  data: u input; y output
function y = fcn(u)
if isnan(u)
    y=0;
else
y = u;
end
end

== matlab function AdaptiveIDMF/ Optical Flow Algorithm for Obstacle Avoidance/Optical flow algorithm and PID Controller for landing/DronePositionEstimation.DroneLandingnoZ/Landing/Subsystem/Subsystem/MATLAB Function ==
  settings: updateMethod=DISCRETE
  data: data input; u input; y output; resetp output
function [y,resetp] = fcn(data, u)
persistent oldd;
persistent resetparam;
persistent param
if isempty(param)
    param=data;
end

if isempty(oldd)
    oldd=u;
end
if isempty(resetparam)
    resetparam=0;
end

if u ==0 || abs(u)>=1
    y=oldd;
    resetparam=resetparam+1;
else
    y=u;

    if resetparam<27
        resetparam=0;
    end
end


oldd = y;
resetp=resetparam;

== matlab function AdaptiveIDMF/ Optical Flow Algorithm for Obstacle Avoidance/Optical flow algorithm and PID Controller for landing/DronePositionEstimation.DroneLandingnoZ/Landing/Subsystem/Subsystem/Varying Gains/variable P/MATLAB Function ==
  settings: updateMethod=DISCRETE
  data: u input; y output; resetparam input
function y = fcn(u, resetparam)
persistent s
if isempty(s)
    s=0;
end
if u>0 && resetparam<16
s=s+0.5;
end
y = s;

== matlab function AdaptiveIDMF/ Optical Flow Algorithm for Obstacle Avoidance/Optical flow algorithm and PID Controller for landing/DronePositionEstimation.DroneLandingnoZ/Landing/Subsystem/Subsystem1/MATLAB Function1 ==
  data: currentz input; y output size=[1,6]; calc input size=6; currentreset input; trainedModel parameter
function y  = fcn(currentz, calc, currentreset,trainedModel)

% persistent mdl
% % 
% if isempty(mdl)
% %    mdl = loadLearnerForCoder('mymdl');
% mdl=0;
% end

y=ones(1,6);
% calcz=calc(1,1);
% ypmin=calc;
% if (currentz-calcz)<=0.03
%     r= 9:1:31;
%     r1= 9:1:31;
%     [r1a,ra]=ndgrid(r1,r);
%     % X=[2*ones(length(r),1),r1,1*ones(length(r),1),1*ones(length(r),1),r];
%     z=(calcz-0.25);
%     X=[z*ones(length(ra(:)),1),ra(:),1*ones(length(ra(:)),1),1*ones(length(ra(:)),1),r1a(:)];
% %     yfit = trainedModel.predictFcn(X);
%     yfit=predict(mdl,X);
%     ypred=[X,yfit];
%     
%     iypreds=find(ypred(:,6)==3);
%     if isempty(iypreds)
%         iypreds=find(ypred(:,6)==2);
%     end
%     ypreds=ypred(iypreds,:);
%     
%     n=min(ypreds(:,2)+ypreds(:,5)); 
%     
%     iypredmin=ypreds(:,2)+ypreds(:,5)<=n+1;
%     ypredmin=ypreds(iypredmin,:);
%     [~,I]=sort(ypredmin(:,2)+ypredmin(:,5));
%     ypredmin=ypredmin(I,:);
%     % r2 = round((d-c).*rand(100,1) + c);
%     % r3=round((d-c).*rand(100,1) + c);
%     r2=1:0.5:20;
%     r3=1:0.5:20;
%     [r2a,r3a]=ndgrid(r2,r3);
%     % X1=[2*ones(length(r2),1),ypredmin(1,2)*ones(length(r2),1),r2,r3,ypredmin(1,5)*ones(length(r1),1)];
%     X1=[z*ones(length(r2a(:)),1),ypredmin(1,2)*ones(length(r2a(:)),1),r2a(:),r3a(:),ypredmin(1,5)*ones(length(r2a(:)),1)];
%     yfit = predict(mdl,X1);
%     yp=[X1,yfit];
%     
%     iyps=find(yp(:,6)==3);
%     if isempty(iyps)
%         iyps=find(yp(:,6)==2);
%     end
%     yps=yp(iyps,:);
%     
%     n1=min(yps(:,3)+yps(:,4)); 
%     
%     iypmin=yps(:,3)+yps(:,4)==n1;
%     ypmin=yps(iypmin,:);
% end
% y = ypmin;
end

== matlab function AdaptiveIDMF/ Optical Flow Algorithm for Obstacle Avoidance/Matlab Function1 ==
  data: ypmin input size=[1,6]; y output size=[1,6]; currentz input; resetparam input; class output
function [y,class] = classifier(ypmin,currentz,resetparam)%#codegen

persistent Mdl
if isempty(Mdl)
   Mdl = loadLearnerForCoder('Model');
end
persistent paramoutput
if isempty(paramoutput)
   paramoutput=ypmin;
end


class=paramoutput(6);
calcz=paramoutput(1,1);


% if (currentz-calcz)<=0.1 && resetparam>=0
if ((currentz-calcz)<=0.1 || currentz < calcz )&& resetparam<=ypmin(5) && resetparam>=0 
    r= 10:1:30;
    r1= 10:1:30;
    [r1a,ra]=ndgrid(r1,r);
    X=[(currentz-0.1)*ones(length(ra(:)),1),ra(:),paramoutput(3)*ones(length(ra(:)),1),paramoutput(4)*ones(length(ra(:)),1),r1a(:)];

%     xm=[(calcz-0.5),paramoutput(2),paramoutput(3),paramoutput(4),paramoutput(5)];
    cout=predict(Mdl,X);
    foutput=[X,cout];

    ifo=find(foutput(:,6)==3);
    if isempty(foutput)
        ifo=find(foutput(:,6)==2);
    end
    if isempty(ifo)
        ifo=find(foutput(:,6)==1);
    end
    foutput1=foutput(ifo,:);
% 
%     n=min(foutput1(:,2)+foutput1(:,5)); 
% 
%     iypredmin=find(foutput1(:,2)+foutput1(:,5)<=n);
%     foutput1=foutput1(iypredmin,:);
%     [p,I]=sort(foutput1(:,2)+foutput1(:,5));
%     foutput1=foutput1(I,:);
    
    r2=2:0.5:20;
    r3=2:0.5:20;
    [r2a,r3a]=ndgrid(r2,r3);
    X1=[(currentz-0.1)*ones(length(r2a(:)),1),foutput1(1,2)*ones(length(r2a(:)),1),r2a(:),r3a(:),foutput1(1,5)*ones(length(r2a(:)),1)];
    cout=predict(Mdl,X1);

    yp=[X1,cout];

    iyps=find(yp(:,6)==3);
    if isempty(iyps)
        iyps=find(yp(:,6)==2);
    end
    yps=yp(iyps,:);
    
%     n1=min(yps(:,3)+yps(:,4)); 
%     
%     iypmin=find(yps(:,3)+yps(:,4)==n1);
%     yps=yps(iypmin,:);
    paramoutput=yps(1,:);
    class=paramoutput(1,6);
end

y = paramoutput;
